simulink model "punkt2"  (R2015b)
settings: Solver=VariableStepAuto  StartTime=0.0  StopTime=30  MaxStep=0.001  MinStep=0.0001  RelTol=1e-3
settings Model: Creator=hohotulca  LastModifiedBy=hohotulca

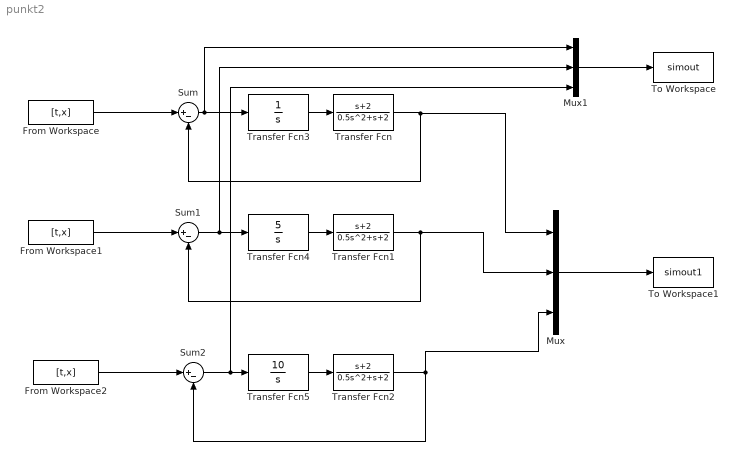
== system punkt2 ==
  From Workspace : FromWorkspace  VariableName=[t,x]  SampleTime=0
  From Workspace1 : FromWorkspace  VariableName=[t,x]  SampleTime=0
  From Workspace2 : FromWorkspace  VariableName=[t,x]  SampleTime=0
  Mux : Mux  Inputs=3
  Mux1 : Mux  Inputs=3
  Sum : Sum  Inputs=|+-
  Sum1 : Sum  Inputs=|+-
  Sum2 : Sum  Inputs=|+-
  To Workspace : ToWorkspace  VariableName=simout  SaveFormat=Timeseries  SampleTime=-1
  To Workspace1 : ToWorkspace  VariableName=simout1  SaveFormat=Timeseries  SampleTime=-1
  Transfer Fcn : TransferFcn  Numerator=[1 2]  Denominator=[0.5 1 2]
  Transfer Fcn1 : TransferFcn  Numerator=[1 2]  Denominator=[0.5 1 2]
  Transfer Fcn2 : TransferFcn  Numerator=[1 2]  Denominator=[0.5 1 2]
  Transfer Fcn3 : TransferFcn  Denominator=[1 0]
  Transfer Fcn4 : TransferFcn  Numerator=[5]  Denominator=[1 0]
  Transfer Fcn5 : TransferFcn  Numerator=[10]  Denominator=[1 0]
  wires:
  Transfer Fcn/1 -> Mux/1, Sum/2
  From Workspace/1 -> Sum/1
  Transfer Fcn1/1 -> Sum1/2, Mux/2
  From Workspace1/1 -> Sum1/1
  Sum1/1 -> Transfer Fcn4/1, Mux1/2
  Transfer Fcn2/1 -> Mux/3, Sum2/2
  From Workspace2/1 -> Sum2/1
  Sum2/1 -> Mux1/3, Transfer Fcn5/1
  Mux/1 -> To Workspace1/1
  Sum/1 -> Transfer Fcn3/1, Mux1/1
  Mux1/1 -> To Workspace/1
  Transfer Fcn3/1 -> Transfer Fcn/1
  Transfer Fcn4/1 -> Transfer Fcn1/1
  Transfer Fcn5/1 -> Transfer Fcn2/1
